simulink model "Datacentre"  (R2026a)
settings: Solver=VariableStepAuto
settings Model: Creator=ragno  LastModifiedBy=ragno

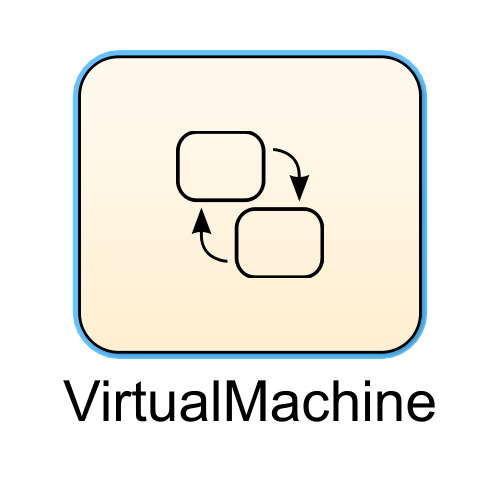
[thumbnail: Simulink's stored preview of the top-level diagram]
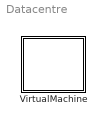
== system Datacentre ==
  VirtualMachine : Stateflow chart  TreatAsAtomicUnit=on

== stateflow chart Datacentre/VirtualMachine ==
  state PoweredOff
  state PoweringOn
  state Resetting
  state PoweringOff
  state PoweredOn
  state Suspending
  state Resuming
  state Suspended
  (default) -> PoweredOff
  PoweringOff -> PoweredOff
  Resetting -> PoweredOn
  PoweredOff -> PoweringOn : PowerOn
  PoweredOn -> Resetting [order 3] : Reset
  PoweringOn -> PoweredOn
  PoweredOn -> PoweringOff [order 1] : PowerOff
  Resuming -> PoweredOn
  PoweredOn -> Suspending [order 2] : Suspend
  Suspending -> Suspended
  Suspended -> Resuming : Resume
  events: PowerOn local FUNCTION_CALL_EVENT; PowerOff local FUNCTION_CALL_EVENT; Suspend local FUNCTION_CALL_EVENT; Resume local FUNCTION_CALL_EVENT; Reset local FUNCTION_CALL_EVENT
